simulink model "motor_4"  (R2023a)
settings: Solver=ode15s  StartTime=0.0  StopTime=sim_end_time  MaxStep=0.0001  RelTol=1e-3
values from neighbouring files (symbols this model uses):
  alpha_cu = 3.9 *10^-3    (= 0.0039)    [BLDC_Motor_params_03.m]    (also in DC_Motor_params_01.m; DC_Motor_params_02.m; DC_Motor_params_04.m; DC_Motor_params_05.m)
  b_m4 = .3    (= 0.3)    [DC_Motor_params_04.m]
  C_t4 = tao_ts_amb_4/res_term_4    (= 92.0668058455)    [DC_Motor_params_04.m]
  ENABLE_SATURATIONS = 1    [run_flags.m]
  ENABLE_SENSORS = 1    [run_flags.m]
  J_eq4 = enc_J_4 + J_r4 + J_4 + 1/8 * m_4 * d_4^2 / r_4^2    [DC_Motor_params_04.m]
  K_d4 = 0    [PID_tuning.m]
  k_e4 = 0.0156    [DC_Motor_params_04.m]
  K_i4 = 0    [PID_tuning.m]
  K_p4 = 2.44    [PID_tuning.m]
  k_t4 = 0.0156    [DC_Motor_params_04.m]
  L_a4 = 0.0336*10^-3    (= 3.36e-05)    [DC_Motor_params_04.m]
  pitch_4 = 0.25    [DC_Motor_params_04.m]
  r_4 = 51    [DC_Motor_params_04.m]
  r_a4_20 = 0.108    [DC_Motor_params_04.m]
  res_term_4 = 9.58    [DC_Motor_params_04.m]
  T_s4_0 = ans.simulationOut.data(end,3)    [use_solo_motor_4.m]
  theta_m4_0 = ans.simulationOut.data(end,1)    [use_solo_motor_4.m]
  voltage_4 = 12    [DC_Motor_params_04.m]
settings Model: Creator=Usuario  LastModifiedBy=Usuario
settings DataIOCC: ExternalInput=[sim_t, sim_data_in]  LoadExternalInput=on

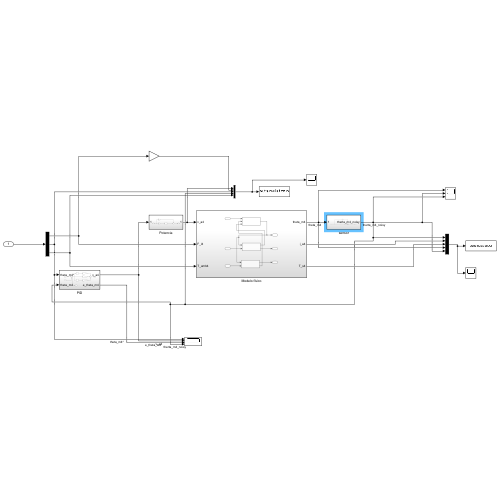
[thumbnail: Simulink's stored preview of the top-level diagram]
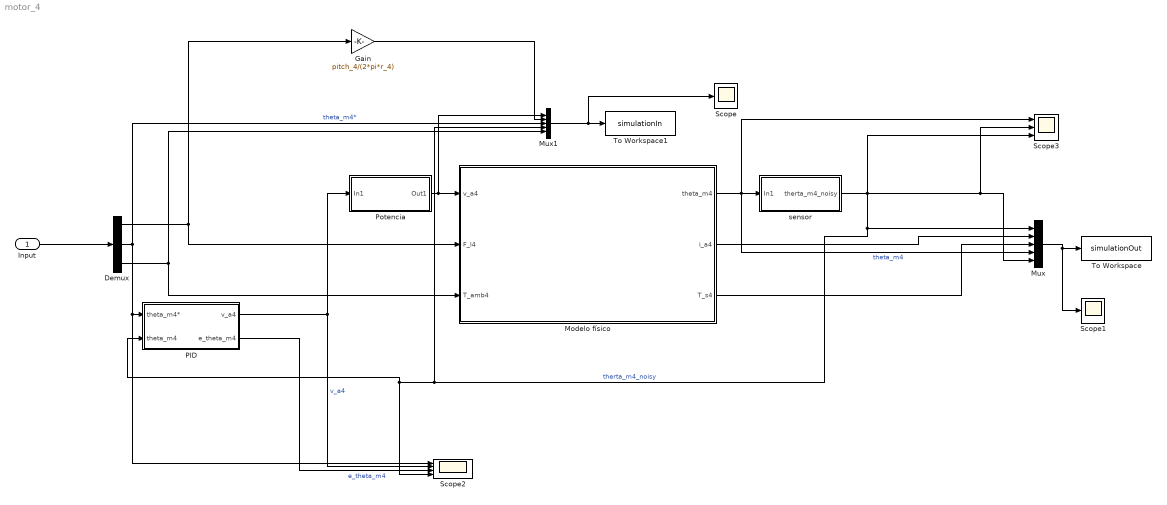
== system motor_4 ==
  Input : Inport
  Demux : Demux  Outputs=3
  Gain : Gain  Gain=pitch_4/(2*pi*r_4)
  Modelo físico : Subsystem
  Mux : Mux  Inputs=5
  Mux1 : Mux  Inputs=5
  PID : Subsystem
  Potencia : Subsystem
  Scope : Scope
  Scope1 : Scope
  Scope2 : Scope  NumInputPorts=4
  Scope3 : Scope  NumInputPorts=3
  To Workspace : ToWorkspace  VariableName=simulationOut  SaveFormat=Timeseries  SampleTime=-1
  To Workspace1 : ToWorkspace  VariableName=simulationIn  SaveFormat=Timeseries  SampleTime=-1
  sensor : Subsystem
  wires:
  Modelo físico/3(T_s4) -> Mux/3
  Demux/2 -> Scope2/1, PID/1(theta_m4*), Mux1/3  "theta_m4*"
  Demux/3 -> Modelo físico/3(T_amb4), Mux1/5
  Input/1 -> Demux/1
  PID/2(e_theta_m4) -> Scope2/3  "e_theta_m4"
  PID/1(v_a4) -> Scope2/2, Potencia/1(In1)  "v_a4"
  Modelo físico/2(i_a4) -> Mux/2
  Mux1/1 -> Scope/1, To Workspace1/1
  Demux/1 -> Modelo físico/2(F_l4), Gain/1
  Mux/1 -> Scope1/1, To Workspace/1
  Modelo físico/1(theta_m4) -> Scope3/1, Mux/4, sensor/1(In1)  "theta_m4"
  Potencia/1(Out1) -> Mux1/1, Modelo físico/1(v_a4)
  Gain/1 -> Mux1/2
  sensor/1(therta_m4_noisy) -> Scope3/2, Mux/5, Scope3/3, Scope2/4, PID/2(theta_m4), Mux1/4, Mux/1  "therta_m4_noisy"

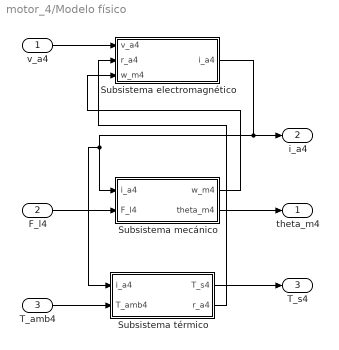
== system motor_4/Modelo físico ==
  v_a4 : Inport
  F_l4 : Inport  Port=2
  T_amb4 : Inport  Port=3
  Subsistema electromagnético : Subsystem
  Subsistema mecánico : Subsystem
  Subsistema térmico : Subsystem
  theta_m4 : Outport
  i_a4 : Outport  Port=2
  T_s4 : Outport  Port=3
  wires:
  Subsistema mecánico/2(theta_m4) -> theta_m4/1
  Subsistema electromagnético/1(i_a4) -> Subsistema térmico/1(i_a4), Subsistema mecánico/1(i_a4), i_a4/1
  v_a4/1 -> Subsistema electromagnético/1(v_a4)
  F_l4/1 -> Subsistema mecánico/2(F_l4)
  Subsistema mecánico/1(w_m4) -> Subsistema electromagnético/3(w_m4)
  T_amb4/1 -> Subsistema térmico/2(T_amb4)
  Subsistema térmico/1(T_s4) -> T_s4/1
  Subsistema térmico/2(r_a4) -> Subsistema electromagnético/2(r_a4)

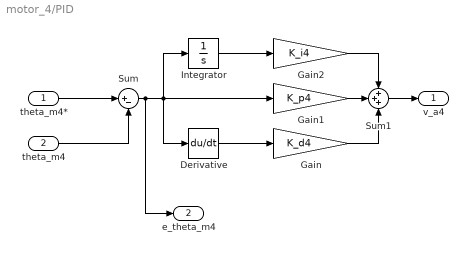
== system motor_4/PID ==
  theta_m4* : Inport
  theta_m4 : Inport  Port=2
  Derivative : Derivative
  Gain : Gain  Gain=K_d4
  Gain1 : Gain  Gain=K_p4
  Gain2 : Gain  Gain=K_i4
  Integrator : Integrator
  Sum : Sum  Inputs=|+-
  Sum1 : Sum  Inputs=+++
  v_a4 : Outport
  e_theta_m4 : Outport  Port=2
  wires:
  theta_m4*/1 -> Sum/1
  theta_m4/1 -> Sum/2
  Sum/1 -> e_theta_m4/1, Integrator/1, Gain1/1, Derivative/1
  Integrator/1 -> Gain2/1
  Derivative/1 -> Gain/1
  Gain1/1 -> Sum1/2
  Gain2/1 -> Sum1/1
  Sum1/1 -> v_a4/1
  Gain/1 -> Sum1/3

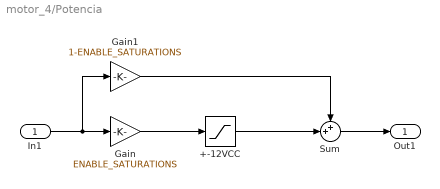
== system motor_4/Potencia ==
  In1 : Inport
  +-12VCC : Saturate  UpperLimit=voltage_4  LowerLimit=-voltage_4
  Gain : Gain  Gain=ENABLE_SATURATIONS
  Gain1 : Gain  Gain=1-ENABLE_SATURATIONS
  Sum : Sum  Inputs=++|
  Out1 : Outport
  wires:
  In1/1 -> Gain1/1, Gain/1
  +-12VCC/1 -> Sum/2
  Gain/1 -> +-12VCC/1
  Sum/1 -> Out1/1
  Gain1/1 -> Sum/1

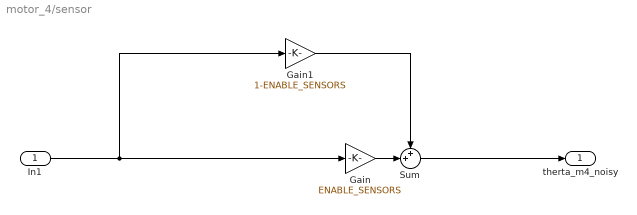
== system motor_4/sensor ==
  In1 : Inport
  Gain : Gain  Gain=ENABLE_SENSORS
  Gain1 : Gain  Gain=1-ENABLE_SENSORS
  Sum : Sum  Inputs=++|
  therta_m4_noisy : Outport
  wires:
  Gain/1 -> Sum/2
  Gain1/1 -> Sum/1
  In1/1 -> Gain/1, Gain1/1
  Sum/1 -> therta_m4_noisy/1

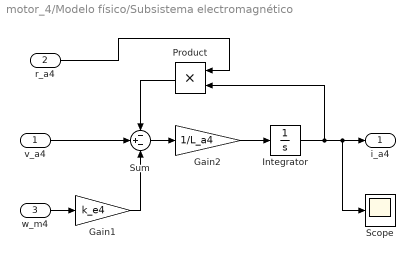
== system motor_4/Modelo físico/Subsistema electromagnético ==
  v_a4 : Inport
  r_a4 : Inport  Port=2
  w_m4 : Inport  Port=3
  Gain1 : Gain  Gain=k_e4
  Gain2 : Gain  Gain=1/L_a4
  Integrator : Integrator
  Product : Product
  Scope : Scope
  Sum : Sum  Inputs=-+-
  i_a4 : Outport
  wires:
  v_a4/1 -> Sum/2
  Integrator/1 -> Product/2, Scope/1, i_a4/1
  Product/1 -> Sum/1
  w_m4/1 -> Gain1/1
  Gain1/1 -> Sum/3
  Sum/1 -> Gain2/1
  Gain2/1 -> Integrator/1
  r_a4/1 -> Product/1

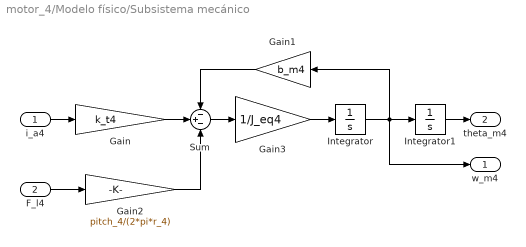
== system motor_4/Modelo físico/Subsistema mecánico ==
  i_a4 : Inport
  F_l4 : Inport  Port=2
  Gain : Gain  Gain=k_t4
  Gain1 : Gain  Gain=b_m4
  Gain2 : Gain  Gain=pitch_4/(2*pi*r_4)
  Gain3 : Gain  Gain=1/J_eq4
  Integrator : Integrator
  Integrator1 : Integrator  InitialCondition=theta_m4_0
  Sum : Sum  Inputs=-+-
  w_m4 : Outport
  theta_m4 : Outport  Port=2
  wires:
  i_a4/1 -> Gain/1
  Gain/1 -> Sum/2
  Integrator/1 -> w_m4/1, Gain1/1, Integrator1/1
  Gain1/1 -> Sum/1
  F_l4/1 -> Gain2/1
  Gain3/1 -> Integrator/1
  Sum/1 -> Gain3/1
  Integrator1/1 -> theta_m4/1
  Gain2/1 -> Sum/3

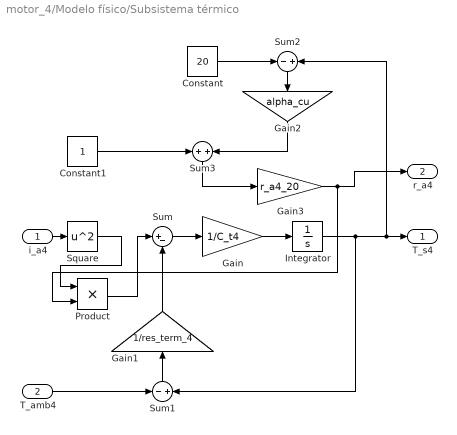
== system motor_4/Modelo físico/Subsistema térmico ==
  i_a4 : Inport
  T_amb4 : Inport  Port=2
  Constant : Constant  Value=20
  Constant1 : Constant
  Gain : Gain  Gain=1/C_t4
  Gain1 : Gain  Gain=1/res_term_4
  Gain2 : Gain  Gain=alpha_cu
  Gain3 : Gain  Gain=r_a4_20
  Integrator : Integrator  InitialCondition=T_s4_0
  Product : Product
  Square : Math  Operator=square
  Sum : Sum  Inputs=|+-
  Sum1 : Sum  Inputs=-|+
  Sum2 : Sum  Inputs=-|+
  Sum3 : Sum  Inputs=+|+
  T_s4 : Outport
  r_a4 : Outport  Port=2
  wires:
  i_a4/1 -> Square/1
  Sum3/1 -> Gain3/1
  Gain2/1 -> Sum3/2
  Square/1 -> Product/1
  Gain3/1 -> Product/2, r_a4/1
  Sum2/1 -> Gain2/1
  T_amb4/1 -> Sum1/1
  Constant1/1 -> Sum3/1
  Gain/1 -> Integrator/1
  Sum/1 -> Gain/1
  Integrator/1 -> Sum1/2, Sum2/2, T_s4/1
  Constant/1 -> Sum2/1
  Sum1/1 -> Gain1/1
  Gain1/1 -> Sum/2
  Product/1 -> Sum/1
